simulink model "i_state_space"  (R2024b)
settings: Solver=VariableStepAuto  StartTime=0.0  StopTime=10.0  RelTol=1e-3
settings Model: Creator=Hp  LastModifiedBy=Hp

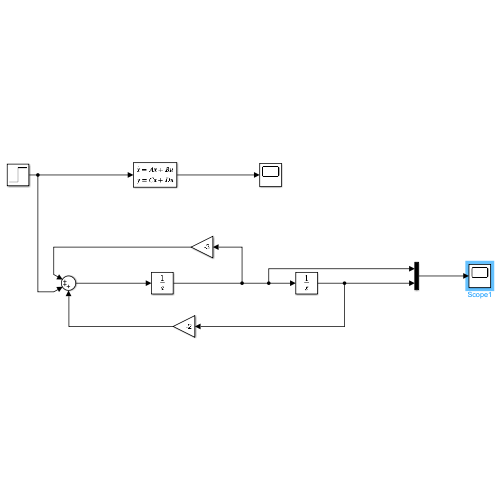
[thumbnail: Simulink's stored preview of the top-level diagram]
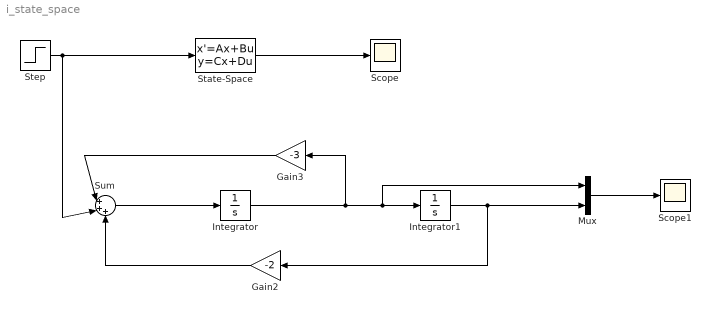
== system i_state_space ==
  Gain2 : Gain  Gain=-2
  Gain3 : Gain  Gain=-3
  Integrator : Integrator
  Integrator1 : Integrator
  Mux : Mux  Inputs=2
  Scope : Scope
  Scope1 : Scope
  State-Space : StateSpace  A=[0 1; -2 -3]  B=[0; 1]  C=[1 0]  D=0  InitialCondition=[0; 0]
  Step : Step  Time=0  SampleTime=0
  Sum : Sum  Inputs=|+++
  wires:
  Step/1 -> Sum/2, State-Space/1
  State-Space/1 -> Scope/1
  Sum/1 -> Integrator/1
  Mux/1 -> Scope1/1
  Gain2/1 -> Sum/3
  Integrator1/1 -> Gain2/1, Mux/2
  Gain3/1 -> Sum/1
  Integrator/1 -> Gain3/1, Mux/1, Integrator1/1
